simulink model "simulatore_non_lineare"  (R2025b)
settings: Solver=VariableStepAuto  StartTime=0.0  StopTime=5  RelTol=1e-3
values from neighbouring files (symbols this model uses):
  C = [C1 C2]    [controllo_scaldatore_elettrico.m]
  u_e = (h_R*A_R)*(x_e(1) - x_e(2))*(1 + K*x_e(1))    [controllo_scaldatore_elettrico.m]
  x_e = [T_R_e; T_out_e]    [controllo_scaldatore_elettrico.m]
libraries: cstblocks x1
settings Model: Creator=39392  LastModifiedBy=39392

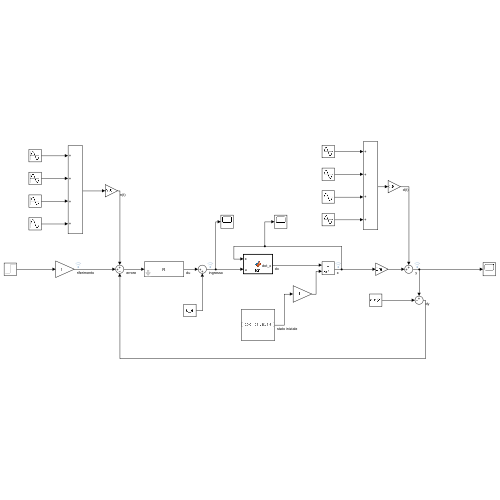
[thumbnail: Simulink's stored preview of the top-level diagram]
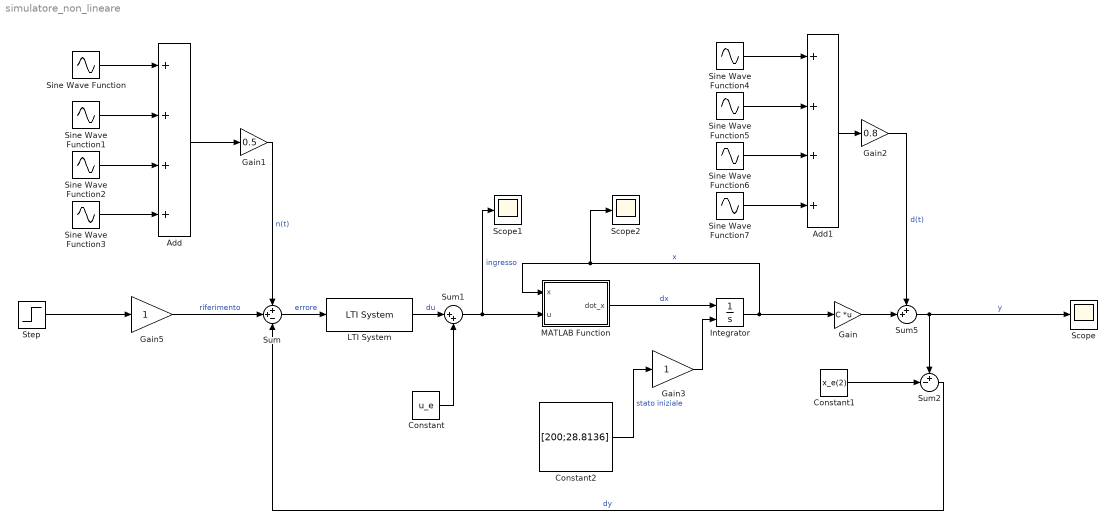
== system simulatore_non_lineare ==
  Add : Sum  Inputs=++++
  Add1 : Sum  Inputs=++++
  Constant : Constant  Value=u_e
  Constant1 : Constant  Value=x_e(2)
  Constant2 : Constant  Value=[200;28.8136]
  Gain : Gain  Gain=C  Multiplication=Matrix(K*u)
  Gain1 : Gain  Gain=0.5
  Gain2 : Gain  Gain=0.8
  Gain3 : Gain
  Gain5 : Gain
  Integrator : Integrator  InitialConditionSource=external  InitialCondition=[200;28.8136]
  LTI System : cstblocks/LTI System  sys=R  IC=[]  PadeOrder=0
  MATLAB Function : MATLAB Function  TreatAsAtomicUnit=on
  Scope : Scope
      settings: ActiveDisplayYMinimum=21.260500036433289  ActiveDisplayYMaximum=96.791499672100443
  Scope1 : Scope
  Scope2 : Scope
      settings: DataLoggingVariableName=ScopeData2
  Sine Wave Function : Sin  Frequency=10^5  SampleTime=0
  Sine Wave Function1 : Sin  Frequency=2*10^5  SampleTime=0
  Sine Wave Function2 : Sin  Frequency=3*10^5  SampleTime=0
  Sine Wave Function3 : Sin  Frequency=4*10^5  SampleTime=0
  Sine Wave Function4 : Sin  Frequency=0.02  SampleTime=0
  Sine Wave Function5 : Sin  Frequency=0.04  SampleTime=0
  Sine Wave Function6 : Sin  Frequency=0.06  SampleTime=0
  Sine Wave Function7 : Sin  Frequency=0.08  SampleTime=0
  Step : Step  After=50  SampleTime=0
  Sum : Sum  Inputs=++-
  Sum1 : Sum  Inputs=|++
  Sum2 : Sum  Inputs=+-|
  Sum5 : Sum  Inputs=++|
  wires:
  Sum/1 -> LTI System/1  "errore"
  LTI System/1 -> Sum1/1  "du"
  Constant/1 -> Sum1/2
  Sum1/1 -> Scope1/1, MATLAB Function/2(u)  "ingresso"
  MATLAB Function/1(dot_x) -> Integrator/1  "dx"
  Integrator/1 -> Scope2/1, MATLAB Function/1(x), Gain/1  "x"
  Constant1/1 -> Sum2/2
  Sum2/1 -> Sum/3  "dy"
  Add/1 -> Gain1/1
  Gain1/1 -> Sum/1  "n(t)"
  Gain/1 -> Sum5/2
  Sum5/1 -> Sum2/1, Scope/1  "y"
  Gain3/1 -> Integrator/2
  Constant2/1 -> Gain3/1  "stato iniziale"
  Sine Wave Function/1 -> Add/1
  Sine Wave Function1/1 -> Add/2
  Sine Wave Function2/1 -> Add/3
  Sine Wave Function3/1 -> Add/4
  Sine Wave Function4/1 -> Add1/1
  Sine Wave Function5/1 -> Add1/2
  Sine Wave Function6/1 -> Add1/3
  Sine Wave Function7/1 -> Add1/4
  Add1/1 -> Gain2/1
  Gain5/1 -> Sum/2  "riferimento"
  Step/1 -> Gain5/1
  Gain2/1 -> Sum5/1  "d(t)"

== matlab function simulatore_non_lineare/MATLAB Function ==
  data: x input; u input; dot_x output
function dot_x = fcn(x,u)

% parametri del sistema
h_R   = 50;          %  coefficiente di convezione tra riscaldatore e aria [W/(m2 C°)]
A_R   = 0.09;        %  area di scambio termico tra riscaldatore e aria [m2]
c_R   = 823.6;       %  calore specifico del riscaldatore [J/(kg C°)]
c_A   = 1010;        %  calore specifico dell'aria [J/(kg C°)]
m_R   = 1.542;       %  massa del riscaldatore [kg];
m_A   = 0.1041;      %  massa dell'aria [kg]
m_A_dot = 0.2;       %  portata massica dell'aria [kg/s].
T_in    = 25;        %  temperatura dell'aria in ingresso (costante) [C°]
K   = 2*10^-3;          %  coefficiente di variazione della resistenza con la temperatura  [1/C°]

dot_x = zeros(2,1);

dot_x(1) = ((h_R*A_R)/(m_R*c_R))*x(2)-((h_R*A_R)/(m_R*c_R))*x(1)+(u/(m_R*c_R)/(1+K*x(1)));
dot_x(2) =  (m_A_dot/m_A)*T_in-((m_A_dot/m_A)+((h_R*A_R)/(m_A*c_A)))*x(2)+((h_R*A_R)/(m_A*c_A))*x(1);
